simulink library "roller485lib"  (R2023a)
settings: Solver=VariableStepAuto  StartTime=0.0  StopTime=10.0  RelTol=1e-3
libraries: arduinolib x172, simulink x66, $bdroot x1
(part 1 of 5)
settings Model: Creator=kawata  LastModifiedBy=kawata
settings RTWCC: GPUComputeCapability=5.0

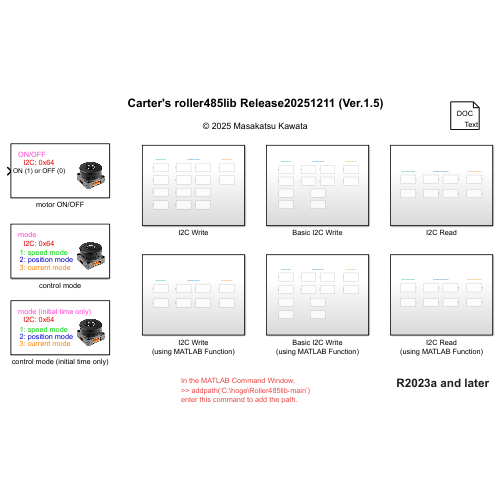
[thumbnail: Simulink's stored preview of the top-level diagram]
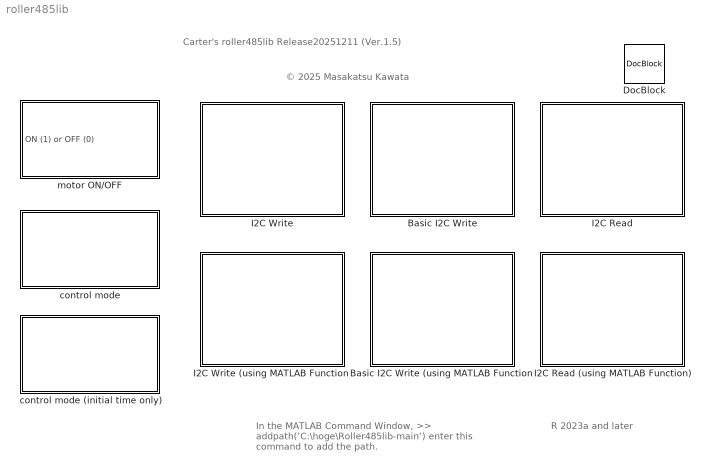
== system roller485lib ==
  note: © 2025 Masakatsu Kawata
  note: Carter's roller485lib Release20251211 (Ver.1.5)
  note: R 2023a and later
  note: In the MATLAB Command Window,
      | >> addpath(‘C:\hoge\Roller485lib-main’)
      | enter this command to add the path.
  Basic I2C Write : Subsystem
  Basic I2C Write (using MATLAB Function) : Subsystem
  DocBlock : simulink/Model-Wide Utilities/DocBlock  DocumentType=Text
      content=|
      | Carter's Roller485lib Ver.1.0
      | Copyright (c) 2025 Masakatsu Kawata
      | Released under the MIT License.
      | See LICENSE for details.
  I2C Read : Subsystem
  I2C Read (using MATLAB Function) : Subsystem
  I2C Write : Subsystem
  I2C Write (using MATLAB Function) : Subsystem
  control mode : Subsystem  mask{I2CAddress=0x64, control_mode=1}
      mask prompts: I2CAddress "I2C Address"; control_mode "mode"
      mask help:
      | 1: speed mode (default)
      | 2: position mode
      | 3: current mode
      | 4: encoder mode
      mask DialogControl ParameterGroupVar Prompt: パラメーター
      mask Display:
      | image('roller485.png', [55,10,75,56]);
      | color('magenta');
      | text(10, 60, 'mode');
      | color('green');
      | text(12, 35, '1: speed mode');
      | color('blue');
      | text(12, 25, '2: position mode');
      | color('orange');
      | text(12, 15, '3: current mode');
      | 
      | color('red');
      | addr = get_param(gcb, 'I2CAddress');
      | text(17, 48, ['I2C: ' addr]);
  control mode (initial time only) : Subsystem  mask{I2CAddress=0x64, control_mode=1}
      mask prompts: I2CAddress "I2C Address"; control_mode "mode"
      mask help:
      | 1: speed mode (default)
      | 2: position mode
      | 3: current mode
      | 4: encoder mode
      | ---------------------------------
      | valid only at the initial time
      mask DialogControl ParameterGroupVar Prompt: パラメーター
      mask Display:
      | image('roller485.png', [55,10,75,56]);
      | color('magenta');
      | text(10, 60, 'mode (initial time only)');
      | color('green');
      | text(12, 35, '1: speed mode');
      | color('blue');
      | text(12, 25, '2: position mode');
      | color('orange');
      | text(12, 15, '3: current mode');
      | 
      | color('red');
      | addr = get_param(gcb, 'I2CAddress');
      | text(17, 48, ['I2C: ' addr]);
  motor ON/OFF : Subsystem  mask{I2CAddress=0x64}
      mask prompts: I2CAddress "I2C Address"
      mask help:
      | 0: motor off
      | 1: motor on
      mask DialogControl ParameterGroupVar Prompt: パラメーター
      mask Display:
      | image('roller485.png', [55,10,75,56]);
      | color('magenta');
      | text(10, 60, 'ON/OFF');
      | 
      | color('red');
      | addr = get_param(gcb, 'I2CAddress');
      | text(17, 48, ['I2C: ' addr]);

== system roller485lib/Basic I2C Write ==
  note: speed mode
  note: current mode
  note: position mode
  basic absolute angle command [deg] : Subsystem  mask{I2CAddress=0x64}
      mask prompts: I2CAddress "I2C Address"
      mask DialogControl ParameterGroupVar Prompt: パラメーター
      mask Display:
      | image('roller485.png', [55,10,75,56]);
      | color('blue');
      | text(10, 60, 'absolute position control');
      | 
      | color('red');
      | addr = get_param(gcb, 'I2CAddress');
      | text(17, 48, ['I2C: ' addr]);
  basic absolute angle command [rad] : Subsystem  mask{I2CAddress=0x64}
      mask prompts: I2CAddress "I2C Address"
      mask DialogControl ParameterGroupVar Prompt: パラメーター
      mask Display:
      | image('roller485.png', [55,10,75,56]);
      | color('blue');
      | text(10, 60, 'absolute position control');
      | 
      | color('red');
      | addr = get_param(gcb, 'I2CAddress');
      | text(17, 48, ['I2C: ' addr]);
  basic angular velocity command [rad/s] : Subsystem  mask{I2CAddress=0x64}
      mask prompts: I2CAddress "I2C Address"
      mask DialogControl ParameterGroupVar Prompt: パラメーター
      mask Display:
      | image('roller485.png', [55,10,75,56]);
      | color('green');
      | text(10, 60, 'speed control');
      | 
      | color('red');
      | addr = get_param(gcb, 'I2CAddress');
      | text(17, 48, ['I2C: ' addr]);
  basic angular velocity command [rpm] : Subsystem  mask{I2CAddress=0x64}
      mask prompts: I2CAddress "I2C Address"
      mask DialogControl ParameterGroupVar Prompt: パラメーター
      mask Display:
      | image('roller485.png', [55,10,75,56]);
      | color('green');
      | text(10, 60, 'speed control');
      | 
      | color('red');
      | addr = get_param(gcb, 'I2CAddress');
      | text(17, 48, ['I2C: ' addr]);
  basic current command [A] : Subsystem  mask{I2CAddress=0x64}
      mask prompts: I2CAddress "I2C Address"
      mask DialogControl ParameterGroupVar Prompt: パラメーター
      mask Display:
      | image('roller485.png', [55,10,75,56]);
      | color('orange');
      | text(10, 60, 'current control');
      | 
      | color('red');
      | addr = get_param(gcb, 'I2CAddress');
      | text(17, 48, ['I2C: ' addr]);
  basic current command [mA] : Subsystem  mask{I2CAddress=0x64}
      mask prompts: I2CAddress "I2C Address"
      mask DialogControl ParameterGroupVar Prompt: パラメーター
      mask Display:
      | image('roller485.png', [55,10,75,56]);
      | color('orange');
      | text(10, 60, 'current control');
      | 
      | color('red');
      | addr = get_param(gcb, 'I2CAddress');
      | text(17, 48, ['I2C: ' addr]);
  basic relative angle command [deg] : Subsystem  mask{I2CAddress=0x64, sample_time=0.005}
      mask prompts: I2CAddress "I2C Address"; sample_time "Sample Time"
      mask DialogControl ParameterGroupVar Prompt: パラメーター
      mask Display:
      | image('roller485.png', [55,10,75,56]);
      | color('blue');
      | text(10, 60, 'relative position control');
      | 
      | color('red');
      | addr = get_param(gcb, 'I2CAddress');
      | text(17, 48, ['I2C: ' addr]);
  basic relative angle command [rad] : Subsystem  mask{I2CAddress=0x64, sample_time=0.005}
      mask prompts: I2CAddress "I2C Address"; sample_time "Sample Time"
      mask DialogControl ParameterGroupVar Prompt: パラメーター
      mask Display:
      | image('roller485.png', [55,10,75,56]);
      | color('blue');
      | text(10, 60, 'relative position control');
      | 
      | color('red');
      | addr = get_param(gcb, 'I2CAddress');
      | text(17, 48, ['I2C: ' addr]);
  position PID : Subsystem  mask{I2CAddress=0x64, position_P=15, position_I=0.000003, position_D=400}
      mask prompts: I2CAddress "I2C Address"; position_P "P"; position_I "I"; position_D "D"
      mask help:
      | position mode
      | ---------------------------------
      | default value
      |  P: 15
      |  I: 0.000003
      |  D: 400
      mask DialogControl ParameterGroupVar Prompt: パラメーター
      mask Display:
      | image('roller485.png', [55,10,75,56]);
      | color('blue');
      | text(10, 60, 'position PID');
      | 
      | color('red');
      | addr = get_param(gcb, 'I2CAddress');
      | text(17, 48, ['I2C: ' addr]);
  position PID (within set time) : Subsystem  mask{I2CAddress=0x64, set_time=0, position_P=15, position_I=0.000003, position_D=400}
      mask prompts: I2CAddress "I2C Address"; set_time "Set Time"; position_P "P"; position_I "I"; position_D "D"
      mask help:
      | position mode
      | ---------------------------------
      | default value
      |  P: 15
      |  I: 0.000003
      |  D: 400
      | ---------------------------------
      | If t ≤ set_time, then PID gain can be set.
      mask DialogControl ParameterGroupVar Prompt: パラメーター
      mask Display:
      | image('roller485.png', [55,10,75,56]);
      | color('blue');
      | text(10, 60, 'position PID');
      | text(10, 47, '(within set time)');
      | 
      | color('red');
      | addr = get_param(gcb, 'I2CAddress');
      | text(17, 34, ['I2C: ' addr]);
  speed PID : Subsystem  mask{I2CAddress=0x64, speed_P=15, speed_I=0.0001, speed_D=400}
      mask prompts: I2CAddress "I2C Address"; speed_P "P"; speed_I "I"; speed_D "D"
      mask help:
      | speed mode
      | ---------------------------------
      | default value
      |  P: 15
      |  I: 0.0001
      |  D: 400
      mask DialogControl ParameterGroupVar Prompt: パラメーター
      mask Display:
      | image('roller485.png', [55,10,75,56]);
      | color('green');
      | text(10, 60, 'speed PID');
      | 
      | color('red');
      | addr = get_param(gcb, 'I2CAddress');
      | text(17, 48, ['I2C: ' addr]);
  speed PID (within set time) : Subsystem  mask{I2CAddress=0x64, set_time=0, speed_P=15, speed_I=0.0001, speed_D=400}
      mask prompts: I2CAddress "I2C Address"; set_time "Set Time"; speed_P "P"; speed_I "I"; speed_D "D"
      mask help:
      | speed mode
      | ---------------------------------
      | default value
      |  P: 15
      |  I: 0.0001
      |  D: 400
      | ---------------------------------
      | valid only at the initial time
      | ---------------------------------
      | If t ≤ set_time, then PID gain can be set.
      mask DialogControl ParameterGroupVar Prompt: パラメーター
      mask Display:
      | image('roller485.png', [55,10,75,56]);
      | color('green');
      | text(10, 60, 'speed PID');
      | text(10, 47, '(within set time)');
      | 
      | color('red');
      | addr = get_param(gcb, 'I2CAddress');
      | text(17, 34, ['I2C: ' addr]);

== system roller485lib/Basic I2C Write (using MATLAB Function) ==
  note: position mode
  note: current mode
  note: speed mode
  basic absolute angle command [deg] (using MATLAB Function) : Subsystem  mask{I2CAddress=0x64}
      mask prompts: I2CAddress "I2C Address"
      mask DialogControl ParameterGroupVar Prompt: パラメーター
      mask Display:
      | image('roller485_matlab_fcn.png', [55,10,75,56]);
      | color('blue');
      | text(10, 60, 'absolute position control');
      | 
      | color('red');
      | addr = get_param(gcb, 'I2CAddress');
      | text(17, 48, ['I2C: ' addr]);
  basic absolute angle command [rad] (using MATLAB Function) : Subsystem  mask{I2CAddress=0x64}
      mask prompts: I2CAddress "I2C Address"
      mask DialogControl ParameterGroupVar Prompt: パラメーター
      mask Display:
      | image('roller485_matlab_fcn.png', [55,10,75,56]);
      | color('blue');
      | text(10, 60, 'absolute position control');
      | 
      | color('red');
      | addr = get_param(gcb, 'I2CAddress');
      | text(17, 48, ['I2C: ' addr]);
  basic angular velocity command [rad/s] (using MATLAB Function) : Subsystem  mask{I2CAddress=0x64}
      mask prompts: I2CAddress "I2C Address"
      mask DialogControl ParameterGroupVar Prompt: パラメーター
      mask Display:
      | image('roller485_matlab_fcn.png', [55,10,75,56]);
      | color('green');
      | text(10, 60, 'speed control');
      | 
      | color('red');
      | addr = get_param(gcb, 'I2CAddress');
      | text(17, 48, ['I2C: ' addr]);
  basic angular velocity command [rpm] (using MATLAB Function) : Subsystem  mask{I2CAddress=0x64}
      mask prompts: I2CAddress "I2C Address"
      mask DialogControl ParameterGroupVar Prompt: パラメーター
      mask Display:
      | image('roller485_matlab_fcn.png', [55,10,75,56]);
      | color('green');
      | text(10, 60, 'speed control');
      | 
      | color('red');
      | addr = get_param(gcb, 'I2CAddress');
      | text(17, 48, ['I2C: ' addr]);
  basic current command [A] (using MATLAB Function) : Subsystem  mask{I2CAddress=0x64}
      mask prompts: I2CAddress "I2C Address"
      mask DialogControl ParameterGroupVar Prompt: パラメーター
      mask Display:
      | image('roller485_matlab_fcn.png', [55,10,75,56]);
      | color('orange');
      | text(10, 60, 'current control');
      | 
      | color('red');
      | addr = get_param(gcb, 'I2CAddress');
      | text(17, 48, ['I2C: ' addr]);
  basic current command [mA] (using MATLAB Function) : Subsystem  mask{I2CAddress=0x64}
      mask prompts: I2CAddress "I2C Address"
      mask DialogControl ParameterGroupVar Prompt: パラメーター
      mask Display:
      | image('roller485_matlab_fcn.png', [55,10,75,56]);
      | color('orange');
      | text(10, 60, 'current control');
      | 
      | color('red');
      | addr = get_param(gcb, 'I2CAddress');
      | text(17, 48, ['I2C: ' addr]);
  basic relative angle command [deg] (using MATLAB Function) : Subsystem  mask{I2CAddress=0x64, sample_time=0.005}
      mask prompts: I2CAddress "I2C Address"; sample_time "Sample Time"
      mask DialogControl ParameterGroupVar Prompt: パラメーター
      mask Display:
      | image('roller485_matlab_fcn.png', [55,10,75,56]);
      | color('blue');
      | text(10, 60, 'relative position control');
      | 
      | color('red');
      | addr = get_param(gcb, 'I2CAddress');
      | text(17, 48, ['I2C: ' addr]);
  basic relative angle command [rad] (using MATLAB Function) : Subsystem  mask{I2CAddress=0x64, sample_time=0.005}
      mask prompts: I2CAddress "I2C Address"; sample_time "Sample Time"
      mask DialogControl ParameterGroupVar Prompt: パラメーター
      mask Display:
      | image('roller485_matlab_fcn.png', [55,10,75,56]);
      | color('blue');
      | text(10, 60, 'relative position control');
      | 
      | color('red');
      | addr = get_param(gcb, 'I2CAddress');
      | text(17, 48, ['I2C: ' addr]);
  position PID (using MATLAB Function) : Subsystem  mask{I2CAddress=0x64, position_P=15, position_I=0.000003, position_D=400}
      mask prompts: I2CAddress "I2C Address"; position_P "P"; position_I "I"; position_D "D"
      mask help:
      | position mode
      | ---------------------------------
      | default value
      |  P: 15
      |  I: 0.000003
      |  D: 400
      mask DialogControl ParameterGroupVar Prompt: パラメーター
      mask Display:
      | image('roller485_matlab_fcn.png', [55,10,75,56]);
      | color('blue');
      | text(10, 60, 'position PID');
      | 
      | color('red');
      | addr = get_param(gcb, 'I2CAddress');
      | text(17, 48, ['I2C: ' addr]);
  position PID (within set time) (using MATLAB Function) : Subsystem  mask{I2CAddress=0x64, set_time=0, position_P=15, position_I=0.000003, position_D=400}
      mask prompts: I2CAddress "I2C Address"; set_time "Set Time"; position_P "P"; position_I "I"; position_D "D"
      mask help:
      | position mode
      | ---------------------------------
      | default value
      |  P: 15
      |  I: 0.000003
      |  D: 400
      | ---------------------------------
      | If t ≤ set_time, then PID gain can be set.
      mask DialogControl ParameterGroupVar Prompt: パラメーター
      mask Display:
      | image('roller485_matlab_fcn.png', [55,10,75,56]);
      | color('blue');
      | text(10, 60, 'position PID');
      | text(10, 47, '(within set time)');
      | 
      | color('red');
      | addr = get_param(gcb, 'I2CAddress');
      | text(17, 34, ['I2C: ' addr]);
  speed PID (using MATLAB Function) : Subsystem  mask{I2CAddress=0x64, speed_P=15, speed_I=0.0001, speed_D=400}
      mask prompts: I2CAddress "I2C Address"; speed_P "P"; speed_I "I"; speed_D "D"
      mask help:
      | speed mode
      | ---------------------------------
      | default value
      |  P: 15
      |  I: 0.0001
      |  D: 400
      mask DialogControl ParameterGroupVar Prompt: パラメーター
      mask Display:
      | image('roller485_matlab_fcn.png', [55,10,75,56]);
      | color('green');
      | text(10, 60, 'speed PID');
      | 
      | color('red');
      | addr = get_param(gcb, 'I2CAddress');
      | text(17, 48, ['I2C: ' addr]);
  speed PID (within set time) (using MATLAB Function) : Subsystem  mask{I2CAddress=0x64, set_time=0, speed_P=15, speed_I=0.0001, speed_D=400}
      mask prompts: I2CAddress "I2C Address"; set_time "Set Time"; speed_P "P"; speed_I "I"; speed_D "D"
      mask help:
      | speed mode
      | ---------------------------------
      | default value
      |  P: 15
      |  I: 0.0001
      |  D: 400
      | ---------------------------------
      | If t ≤ set_time, then PID gain can be set.
      mask DialogControl ParameterGroupVar Prompt: パラメーター
      mask Display:
      | image('roller485_matlab_fcn.png', [55,10,75,56]);
      | color('green');
      | text(10, 60, 'speed PID');
      | text(10, 47, '(within set time)');
      | 
      | color('red');
      | addr = get_param(gcb, 'I2CAddress');
      | text(17, 34, ['I2C: ' addr]);

== system roller485lib/I2C Read ==
  note: speed detection
  note: current detection
  note: position detection
  absolute angle detection [deg] : Subsystem  mask{I2CAddress=0x64, sample_time=0.005}
      mask prompts: I2CAddress "I2C Address"; sample_time "Sample Time"
      mask DialogControl ParameterGroupVar Prompt: パラメーター
      mask Display:
      | image('roller485.png', [30,10,75,56]);
      | color('blue');
      | text(10, 60, 'absolute angle detection');
      | 
      | color('red');
      | addr = get_param(gcb, 'I2CAddress');
      | text(17, 48, ['I2C: ' addr]);
  absolute angle detection [rad] : Subsystem  mask{I2CAddress=0x64, sample_time=0.005}
      mask prompts: I2CAddress "I2C Address"; sample_time "Sample Time"
      mask DialogControl ParameterGroupVar Prompt: パラメーター
      mask Display:
      | image('roller485.png', [30,10,75,56]);
      | color('blue');
      | text(10, 60, 'absolute angle detection');
      | 
      | color('red');
      | addr = get_param(gcb, 'I2CAddress');
      | text(17, 48, ['I2C: ' addr]);
  angular velocity detection using LPF [rad/s] : Subsystem  mask{I2CAddress=0x64, sample_time=0.005}
      mask prompts: I2CAddress "I2C Address"; sample_time "Sample Time"
      mask DialogControl ParameterGroupVar Prompt: パラメーター
      mask Display:
      | image('roller485.png', [30,10,75,56]);
      | color('green');
      | text(10, 60, 'speed detection');
      | 
      | color('red');
      | addr = get_param(gcb, 'I2CAddress');
      | text(17, 48, ['I2C: ' addr]);
  angular velocity detection using LPF [rpm] : Subsystem  mask{I2CAddress=0x64, sample_time=0.005}
      mask prompts: I2CAddress "I2C Address"; sample_time "Sample Time"
      mask DialogControl ParameterGroupVar Prompt: パラメーター
      mask Display:
      | image('roller485.png', [30,10,75,56]);
      | color('green');
      | text(10, 60, 'speed detection');
      | 
      | color('red');
      | addr = get_param(gcb, 'I2CAddress');
      | text(17, 48, ['I2C: ' addr]);
  current detection [A] : Subsystem  mask{I2CAddress=0x64, sample_time=0.005}
      mask prompts: I2CAddress "I2C Address"; sample_time "Sample Time"
      mask DialogControl ParameterGroupVar Prompt: パラメーター
      mask Display:
      | image('roller485.png', [30,10,75,56]);
      | color('orange');
      | text(10, 60, 'current detection');
      | 
      | color('red');
      | addr = get_param(gcb, 'I2CAddress');
      | text(17, 48, ['I2C: ' addr]);
  current detection [mA] : Subsystem  mask{I2CAddress=0x64, sample_time=0.005}
      mask prompts: I2CAddress "I2C Address"; sample_time "Sample Time"
      mask DialogControl ParameterGroupVar Prompt: パラメーター
      mask Display:
      | image('roller485.png', [30,10,75,56]);
      | color('orange');
      | text(10, 60, 'current detection');
      | 
      | color('red');
      | addr = get_param(gcb, 'I2CAddress');
      | text(17, 48, ['I2C: ' addr]);
  relative angle detection [deg] : Subsystem  mask{I2CAddress=0x64, sample_time=0.005, set_time=0}
      mask prompts: I2CAddress "I2C Address"; sample_time "Sample Time"; set_time "Set Time"
      mask help: If t ≤ set_time, then initial angle is set.
      mask DialogControl ParameterGroupVar Prompt: パラメーター
      mask Display:
      | image('roller485.png', [30,10,75,56]);
      | color('blue');
      | text(10, 60, 'relative angle detection');
      | 
      | color('red');
      | addr = get_param(gcb, 'I2CAddress');
      | text(17, 48, ['I2C: ' addr]);
  relative angle detection [rad] : Subsystem  mask{I2CAddress=0x64, sample_time=0.005, set_time=0}
      mask prompts: I2CAddress "I2C Address"; sample_time "Sample Time"; set_time "Set Time"
      mask help: If t ≤ set_time, then initial angle is set.
      mask DialogControl ParameterGroupVar Prompt: パラメーター
      mask Display:
      | image('roller485.png', [30,10,75,56]);
      | color('blue');
      | text(10, 60, 'relative angle detection');
      | 
      | color('red');
      | addr = get_param(gcb, 'I2CAddress');
      | text(17, 48, ['I2C: ' addr]);

== system roller485lib/I2C Read (using MATLAB Function) ==
  note: position detection
  note: current detection
  note: speed detection
  absolute angle detection [deg] (using MATLAB Function) : Subsystem  mask{I2CAddress=0x64, sample_time=0.005}
      mask prompts: I2CAddress "I2C Address"; sample_time "Sample Time"
      mask DialogControl ParameterGroupVar Prompt: パラメーター
      mask Display:
      | image('roller485_matlab_fcn.png', [38,10,75,56]);
      | color('blue');
      | text(10, 60, 'absolute angle detection');
      | 
      | color('red');
      | addr = get_param(gcb, 'I2CAddress');
      | text(17, 48, ['I2C: ' addr]);
  absolute angle detection [rad] (using MATLAB Function) : Subsystem  mask{I2CAddress=0x64, sample_time=0.005}
      mask prompts: I2CAddress "I2C Address"; sample_time "Sample Time"
      mask DialogControl ParameterGroupVar Prompt: パラメーター
      mask Display:
      | image('roller485_matlab_fcn.png', [38,10,75,56]);
      | color('blue');
      | text(10, 60, 'absolute angle detection');
      | 
      | color('red');
      | addr = get_param(gcb, 'I2CAddress');
      | text(17, 48, ['I2C: ' addr]);
  angular velocity detection using LPF [rad/s] (using MATLAB Function) : Subsystem  mask{I2CAddress=0x64, sample_time=0.005}
      mask prompts: I2CAddress "I2C Address"; sample_time "Sample Time"
      mask DialogControl ParameterGroupVar Prompt: パラメーター
      mask Display:
      | image('roller485_matlab_fcn.png', [38,10,75,56]);
      | color('green');
      | text(10, 60, 'speed detection');
      | 
      | color('red');
      | addr = get_param(gcb, 'I2CAddress');
      | text(17, 48, ['I2C: ' addr]);
  angular velocity detection using LPF [rpm] (using MATLAB Function) : Subsystem  mask{I2CAddress=0x64, sample_time=0.005}
      mask prompts: I2CAddress "I2C Address"; sample_time "Sample Time"
      mask DialogControl ParameterGroupVar Prompt: パラメーター
      mask Display:
      | image('roller485_matlab_fcn.png', [38,10,75,56]);
      | color('green');
      | text(10, 60, 'speed detection');
      | 
      | color('red');
      | addr = get_param(gcb, 'I2CAddress');
      | text(17, 48, ['I2C: ' addr]);
  current detection [A] (using MATLAB Function) : Subsystem  mask{I2CAddress=0x64, sample_time=0.005}
      mask prompts: I2CAddress "I2C Address"; sample_time "Sample Time"
      mask DialogControl ParameterGroupVar Prompt: パラメーター
      mask Display:
      | image('roller485_matlab_fcn.png', [38,10,75,56]);
      | color('orange');
      | text(10, 60, 'current detection');
      | 
      | color('red');
      | addr = get_param(gcb, 'I2CAddress');
      | text(17, 48, ['I2C: ' addr]);
  current detection [mA] (using MATLAB Function) : Subsystem  mask{I2CAddress=0x64, sample_time=0.005}
      mask prompts: I2CAddress "I2C Address"; sample_time "Sample Time"
      mask DialogControl ParameterGroupVar Prompt: パラメーター
      mask Display:
      | image('roller485_matlab_fcn.png', [38,10,75,56]);
      | color('orange');
      | text(10, 60, 'current detection');
      | 
      | color('red');
      | addr = get_param(gcb, 'I2CAddress');
      | text(17, 48, ['I2C: ' addr]);
  relative angle detection [deg] (using MATLAB Function) : Subsystem  mask{I2CAddress=0x64, sample_time=0.005, set_time=0}
      mask prompts: I2CAddress "I2C Address"; sample_time "Sample Time"; set_time "Set Time"
      mask help: If t ≤ set_time, then initial angle is set.
      mask DialogControl ParameterGroupVar Prompt: パラメーター
      mask Display:
      | image('roller485_matlab_fcn.png', [38,10,75,56]);
      | color('blue');
      | text(10, 60, 'relative angle detection');
      | 
      | color('red');
      | addr = get_param(gcb, 'I2CAddress');
      | text(17, 48, ['I2C: ' addr]);
  relative angle detection [rad] (using MATLAB Function) : Subsystem  mask{I2CAddress=0x64, sample_time=0.005, set_time=0}
      mask prompts: I2CAddress "I2C Address"; sample_time "Sample Time"; set_time "Set Time"
      mask help: If t ≤ set_time, then initial angle is set.
      mask DialogControl ParameterGroupVar Prompt: パラメーター
      mask Display:
      | image('roller485_matlab_fcn.png', [38,10,75,56]);
      | color('blue');
      | text(10, 60, 'relative angle detection');
      | 
      | color('red');
      | addr = get_param(gcb, 'I2CAddress');
      | text(17, 48, ['I2C: ' addr]);

== system roller485lib/I2C Write ==
  note: position mode
  note: current mode
  note: speed mode
  absolute angle command [deg] : Subsystem  mask(absolute angle command [deg]){I2CAddress=0x64, position_P=15, position_I=0.000003, position_D=400, set_time1=0, set_time2=0}
      mask prompts: I2CAddress "I2C Address"; position_P "P"; position_I "I"; position_D "D"; set_time1 "Set Time1"; set_time2 "Set Time2"
      mask help:
      | position mode
      | If t ≤ set_time1, then position mode is set.
      | ---------------------------------
      | default value (PID gain of position controller)
      |  P: 15
      |  I: 0.000003
      |  D: 400
      | If t ≤ set_time2, then PID gain can be set.
      mask DialogControl ParameterGroupVar Prompt: パラメーター
      mask Display:
      | image('roller485.png', [55,10,75,56]);
      | color('blue');
      | text(10, 60, 'absolute position control');
      | text(17, 22, '# mode setting');
      | text(17, 10, '# PID gain setting');
      | color('black');
      | 
      | color('red');
      | addr = get_param(gcb, 'I2CAddress');
      | text(17, 48, ['I2C: ' addr]);
  absolute angle command [deg] and max current [mA] : Subsystem  mask(absolute angle command [deg]){I2CAddress=0x64, position_P=15, position_I=0.000003, position_D=400, max_current=1000, set_time1=0, set_time2=0, set_time3=0}
      mask prompts: I2CAddress "I2C Address"; position_P "P"; position_I "I"; position_D "D"; max_current "Imax [mA]"; set_time1 "Set Time1"; set_time2 "Set Time2"; set_time3 "Set Time3"
      mask help:
      | position mode
      | If t ≤ set_time1, then position mode is set.
      | ---------------------------------
      | default value (PID gain of position controller)
      |  P: 15
      |  I: 0.000003
      |  D: 400
      | If t ≤ set_time2, then PID gain can be set.
      | ---------------------------------
      | default value (Imax: max current)
      |  Imax: 1000 mA
      |   ---> Imax can be set up to a maximum of 1200mA.
      | If t ≤ set_time3, then Imax can be set.
      mask DialogControl ParameterGroupVar Prompt: パラメーター
      mask Display:
      | image('roller485.png', [55,10,75,56]);
      | color('blue');
      | text(10, 60, 'absolute position control');
      | text(17, 22, '# mode setting');
      | text(17, 10, '# PID gain & Imax setting');
      | 
      | color('red');
      | addr = get_param(gcb, 'I2CAddress');
      | text(17, 48, ['I2C: ' addr]);
  absolute angle command [rad] : Subsystem  mask(absolute angle command [rad]){I2CAddress=0x64, position_P=15, position_I=0.000003, position_D=400, set_time1=0, set_time2=0}
      mask prompts: I2CAddress "I2C Address"; position_P "P"; position_I "I"; position_D "D"; set_time1 "Set Time1"; set_time2 "Set Time2"
      mask help:
      | position mode
      | If t ≤ set_time1, then position mode is set.
      | ---------------------------------
      | default value (PID gain of position controller)
      |  P: 15
      |  I: 0.000003
      |  D: 400
      | If t ≤ set_time2, then PID gain can be set.
      mask DialogControl ParameterGroupVar Prompt: パラメーター
      mask Display:
      | image('roller485.png', [55,10,75,56]);
      | color('blue');
      | text(10, 60, 'absolute position control');
      | text(17, 22, '# mode setting');
      | text(17, 10, '# PID gain setting');
      | 
      | color('red');
      | addr = get_param(gcb, 'I2CAddress');
      | text(17, 48, ['I2C: ' addr]);
  absolute angle command [rad] and max current [mA] : Subsystem  mask(absolute angle command [rad]){I2CAddress=0x64, position_P=15, position_I=0.000003, position_D=400, max_current=1000, set_time1=0, set_time2=0, set_time3=0}
      mask prompts: I2CAddress "I2C Address"; position_P "P"; position_I "I"; position_D "D"; max_current "Imax [mA]"; set_time1 "Set Time1"; set_time2 "Set Time2"; set_time3 "Set Time3"
      mask help:
      | position mode
      | If t ≤ set_time1, then position mode is set.
      | ---------------------------------
      | default value (PID gain of position controller)
      |  P: 15
      |  I: 0.000003
      |  D: 400
      | If t ≤ set_time2, then PID gain can be set.
      | ---------------------------------
      | default value (Imax: max current)
      |  Imax: 1000 mA
      |   ---> Imax can be set up to a maximum of 1200mA.
      | If t ≤ set_time3, then Imax can be set.
      mask DialogControl ParameterGroupVar Prompt: パラメーター
      mask Display:
      | image('roller485.png', [55,10,75,56]);
      | color('blue');
      | text(10, 60, 'absolute position control');
      | text(17, 22, '# mode setting');
      | text(17, 10, '# PID gain & Imax setting');
      | 
      | color('red');
      | addr = get_param(gcb, 'I2CAddress');
      | text(17, 48, ['I2C: ' addr]);
  angular velocity command [rad/s] : Subsystem  mask(angular velocity command [rad/s]){I2CAddress=0x64, speed_P=15, speed_I=0.0001, speed_D=400, set_time1=0, set_time2=0}
      mask prompts: I2CAddress "I2C Address"; speed_P "P"; speed_I "I"; speed_D "D"; set_time1 "Set Time1"; set_time2 "Set Time2"
      mask help:
      | speed mode
      | If t ≤ set_time1, then speed mode is set.
      | ---------------------------------
      | default value (PID gain of speed controller)
      |  P: 15
      |  I: 0.0001
      |  D: 400
      | If t ≤ set_time2, then PID gain can be set.
      mask DialogControl ParameterGroupVar Prompt: パラメーター
      mask Display:
      | image('roller485.png', [55,10,75,56]);
      | color('green');
      | text(10, 60, 'speed control');
      | text(17, 22, '# mode setting');
      | text(17, 10, '# PID gain setting');
      | 
      | color('red');
      | addr = get_param(gcb, 'I2CAddress');
      | text(17, 48, ['I2C: ' addr]);
  angular velocity command [rad/s] and max current [mA] : Subsystem  mask(angular velocity command [rad/s]){I2CAddress=0x64, speed_P=15, speed_I=0.0001, speed_D=400, max_current=1000, set_time1=0, set_time2=0, set_time3=0}
      mask prompts: I2CAddress "I2C Address"; speed_P "P"; speed_I "I"; speed_D "D"; max_current "Imax [mA]"; set_time1 "Set Time1"; set_time2 "Set Time2"; set_time3 "Set Time3"
      mask help:
      | speed mode
      | If t ≤ set_time1, then speed mode is set.
      | ---------------------------------
      | default value (PID gain of speed controller)
      |  P: 15
      |  I: 0.0001
      |  D: 400
      | If t ≤ set_time2, then PID gain and Imax can be set.
      | ---------------------------------
      | default value (Imax: max current)
      |  Imax: 1000 mA
      |  ---> Imax can be set up to a maximum of 1200mA.
      | If t ≤ set_time3, then Imax is set.
      mask DialogControl ParameterGroupVar Prompt: パラメーター
      mask Display:
      | image('roller485.png', [55,10,75,56]);
      | color('green');
      | text(10, 60, 'speed control');
      | text(17, 22, '# mode setting');
      | text(17, 10, '# PID gain & Imax setting');
      | 
      | color('red');
      | addr = get_param(gcb, 'I2CAddress');
      | text(17, 48, ['I2C: ' addr]);
  angular velocity command [rpm] : Subsystem  mask(angular velocity command [rpm]){I2CAddress=0x64, speed_P=15, speed_I=0.0001, speed_D=400, set_time1=0, set_time2=0}
      mask prompts: I2CAddress "I2C Address"; speed_P "P"; speed_I "I"; speed_D "D"; set_time1 "Set Time1"; set_time2 "Set Time2"
      mask help:
      | speed mode
      | If t ≤ set_time1, then speed mode is set.
      | ---------------------------------
      | default value (PID gain of speed controller)
      |  P: 15
      |  I: 0.0001
      |  D: 400
      | If t ≤ set_time2, then PID gain can be set.
      mask DialogControl ParameterGroupVar Prompt: パラメーター
      mask Display:
      | image('roller485.png', [55,10,75,56]);
      | color('green');
      | text(10, 60, 'speed control');
      | color('green');
      | text(17, 22, '# mode setting');
      | text(17, 10, '# PID gain setting');
      | 
      | color('red');
      | addr = get_param(gcb, 'I2CAddress');
      | text(17, 48, ['I2C: ' addr]);
  angular velocity command [rpm] and max current [mA] : Subsystem  mask(angular velocity command [rpm]){I2CAddress=0x64, speed_P=15, speed_I=0.0001, speed_D=400, max_current=1000, set_time1=0, set_time2=0, set_time3=0}
      mask prompts: I2CAddress "I2C Address"; speed_P "P"; speed_I "I"; speed_D "D"; max_current "Imax [mA]"; set_time1 "Set Time1"; set_time2 "Set Time2"; set_time3 "Set Time3"
      mask help:
      | speed mode
      | If t ≤ set_time1, then speed mode is set.
      | ---------------------------------
      | default value (PID gain of speed controller)
      |  P: 15
      |  I: 0.0001
      |  D: 400
      | If t ≤ set_time2, then PID gain and Imax can be set.
      | ---------------------------------
      | default value (Imax: max current)
      |  Imax: 1000 mA
      |  ---> Imax can be set up to a maximum of 1200mA.
      | If t ≤ set_time3, then Imax is set.
      mask DialogControl ParameterGroupVar Prompt: パラメーター
      mask Display:
      | image('roller485.png', [55,10,75,56]);
      | color('green');
      | text(10, 60, 'speed control');
      | text(17, 22, '# mode setting');
      | text(17, 10, '# PID gain & Imax setting');
      | 
      | color('red');
      | addr = get_param(gcb, 'I2CAddress');
      | text(17, 48, ['I2C: ' addr]);
  current command [A] : Subsystem  mask(current command [A]){I2CAddress=0x64, set_time=0}
      mask prompts: I2CAddress "I2C Address"; set_time "Set Time"
      mask help:
      | current mode
      | If t ≤ set_time, then current mode is set.
      | ---------------------------------
      | PID gain of current controller
      |  P: 0.002
      |  I: 0.00005
      |  D: 0
      | Changing the PID gains is not permitted.
      mask DialogControl ParameterGroupVar Prompt: パラメーター
      mask Display:
      | image('roller485.png', [55,10,75,56]);
      | color('orange');
      | text(10, 60, 'current control');
      | text(17, 22, '# mode setting');
      | 
      | color('red');
      | addr = get_param(gcb, 'I2CAddress');
      | text(17, 48, ['I2C: ' addr]);
  current command [mA] : Subsystem  mask(current command [A]){I2CAddress=0x64, set_time=0}
      mask prompts: I2CAddress "I2C Address"; set_time "Set Time"
      mask help:
      | current mode
      | If t ≤ set_time, then current mode is set.
      | ---------------------------------
      | PID gain of current controller
      |  P: 0.002
      |  I: 0.00005
      |  D: 0
      | Changing the PID gains is not permitted.
      mask DialogControl ParameterGroupVar Prompt: パラメーター
      mask Display:
      | image('roller485.png', [55,10,75,56]);
      | color('orange');
      | text(10, 60, 'current control');
      | text(17, 22, '# mode setting');
      | 
      | color('red');
      | addr = get_param(gcb, 'I2CAddress');
      | text(17, 48, ['I2C: ' addr]);
  relative angle command [deg] : Subsystem  mask(relative angle command [deg]){I2CAddress=0x64, sample_time=0.005, position_P=15, position_I=0.000003, position_D=400, set_time1=0, set_time2=0}
      mask prompts: I2CAddress "I2C Address"; sample_time "Sample Time"; position_P "P"; position_I "I"; position_D "D"; set_time1 "Set Time1"; set_time2 "Set Time2"
      mask help:
      | position mode
      | If t ≤ set_time1, then position mode and initial angle are set.
      | ---------------------------------
      | default value (PID gain of position controller)
      |  P: 15
      |  I: 0.000003
      |  D: 400
      | If t ≤ set_time2, then PID gain can be set.
      mask DialogControl ParameterGroupVar Prompt: パラメーター
      mask Display:
      | image('roller485.png', [55,10,75,56]);
      | color('blue');
      | text(10, 60, 'relative position control');
      | text(17, 22, '# mode setting');
      | text(17, 10, '# PID gain setting');
      | 
      | color('red');
      | addr = get_param(gcb, 'I2CAddress');
      | text(17, 48, ['I2C: ' addr]);
  relative angle command [deg] and max current [mA] : Subsystem  mask(relative angle command [rad]){I2CAddress=0x64, sample_time=0.005, position_P=15, position_I=0.000003, position_D=400, max_current=1000, set_time1=0, set_time2=0, set_time3=0}
      mask prompts: I2CAddress "I2C Address"; sample_time "Sample Time"; position_P "P"; position_I "I"; position_D "D"; max_current "Imax [mA]"; set_time1 "Set Time1"; set_time2 "Set Time2"; set_time3 "Set Time3"
      mask help:
      | position mode
      | If t ≤ set_time1, then position mode and initial angle are set.
      | ---------------------------------
      | default value (PID gain of position controller)
      |  P: 15
      |  I: 0.000003
      |  D: 400
      | If t ≤ set_time2, then PID gain can be set.
      | ---------------------------------
      | default value (Imax: max current)
      |  Imax: 1000 mA
      |   ---> Imax can be set up to a maximum of 1200mA.
      | If t ≤ set_time3, then Imax can be set.
      mask DialogControl ParameterGroupVar Prompt: パラメーター
      mask Display:
      | image('roller485.png', [55,10,75,56]);
      | color('blue');
      | text(10, 60, 'relative position control');
      | text(17, 22, '# mode setting');
      | text(17, 10, '# PID gain & Imax setting');
      | 
      | color('red');
      | addr = get_param(gcb, 'I2CAddress');
      | text(17, 48, ['I2C: ' addr]);
  relative angle command [rad] : Subsystem  mask(relative angle command [rad]){I2CAddress=0x64, sample_time=0.005, position_P=15, position_I=0.000003, position_D=400, set_time1=0, set_time2=0}
      mask prompts: I2CAddress "I2C Address"; sample_time "Sample Time"; position_P "P"; position_I "I"; position_D "D"; set_time1 "Set Time1"; set_time2 "Set Time2"
      mask help:
      | position mode
      | If t ≤ set_time1, then position mode and initial angle are set.
      | ---------------------------------
      | default value (PID gain of position controller)
      |  P: 15
      |  I: 0.000003
      |  D: 400
      | If t ≤ set_time2, then PID gain can be set.
      mask DialogControl ParameterGroupVar Prompt: パラメーター
      mask Display:
      | image('roller485.png', [55,10,75,56]);
      | color('blue');
      | text(10, 60, 'relative position control');
      | text(17, 22, '# mode setting');
      | text(17, 10, '# PID gain setting');
      | 
      | color('red');
      | addr = get_param(gcb, 'I2CAddress');
      | text(17, 48, ['I2C: ' addr]);
  relative angle command [rad] and max current [mA] : Subsystem  mask(relative angle command [rad]){I2CAddress=0x64, sample_time=0.005, position_P=15, position_I=0.000003, position_D=400, max_current=1000, set_time1=0, set_time2=0, set_time3=0}
      mask prompts: I2CAddress "I2C Address"; sample_time "Sample Time"; position_P "P"; position_I "I"; position_D "D"; max_current "Imax [mA]"; set_time1 "Set Time1"; set_time2 "Set Time2"; set_time3 "Set Time3"
      mask help:
      | position mode
      | If t ≤ set_time1, then position mode and initial angle are set.
      | ---------------------------------
      | default value (PID gain of position controller)
      |  P: 15
      |  I: 0.000003
      |  D: 400
      | If t ≤ set_time2, then PID gain can be set.
      | ---------------------------------
      | default value (Imax: max current)
      |  Imax: 1000 mA
      |   ---> Imax can be set up to a maximum of 1200mA.
      | If t ≤ set_time3, then Imax can be set.
      mask DialogControl ParameterGroupVar Prompt: パラメーター
      mask Display:
      | image('roller485.png', [55,10,75,56]);
      | color('blue');
      | text(10, 60, 'relative position control');
      | text(17, 22, '# mode setting');
      | text(17, 10, '# PID gain & Imax setting');
      | 
      | color('red');
      | addr = get_param(gcb, 'I2CAddress');
      | text(17, 48, ['I2C: ' addr]);

== system roller485lib/I2C Write (using MATLAB Function) ==
  note: speed mode
  note: current mode
  note: position mode
  absolute angle command [deg] (using MATLAB Function) : Subsystem  mask(absolute angle command [deg]){I2CAddress=0x64, position_P=15, position_I=0.000003, position_D=400, set_time1=0, set_time2=0}
      mask prompts: I2CAddress "I2C Address"; position_P "P"; position_I "I"; position_D "D"; set_time1 "Set Time1"; set_time2 "Set Time2"
      mask help:
      | position mode
      | If t ≤ set_time1, then position mode is set.
      | ---------------------------------
      | default value (PID gain of position controller)
      |  P: 15
      |  I: 0.000003
      |  D: 400
      | If t ≤ set_time2, then PID gain can be set.
      mask DialogControl ParameterGroupVar Prompt: パラメーター
      mask Display:
      | image('roller485_matlab_fcn.png', [55,10,75,56]);
      | color('blue');
      | text(10, 60, 'absolute position control');
      | text(17, 22, '# mode setting');
      | text(17, 10, '# PID gain setting');
      | 
      | color('red');
      | addr = get_param(gcb, 'I2CAddress');
      | text(17, 48, ['I2C: ' addr]);
  absolute angle command [rad] (using MATLAB Function) : Subsystem  mask(absolute angle command [rad]){I2CAddress=0x64, position_P=15, position_I=0.000003, position_D=400, set_time1=0, set_time2=0}
      mask prompts: I2CAddress "I2C Address"; position_P "P"; position_I "I"; position_D "D"; set_time1 "Set Time1"; set_time2 "Set Time2"
      mask help:
      | position mode
      | If t ≤ set_time1, then position mode is set.
      | ---------------------------------
      | default value (PID gain of position controller)
      |  P: 15
      |  I: 0.000003
      |  D: 400
      | If t ≤ set_time2, then PID gain can be set.
      mask DialogControl ParameterGroupVar Prompt: パラメーター
      mask Display:
      | image('roller485_matlab_fcn.png', [55,10,75,56]);
      | color('blue');
      | text(10, 60, 'absolute position control');
      | text(17, 22, '# mode setting');
      | text(17, 10, '# PID gain setting');
      | 
      | color('red');
      | addr = get_param(gcb, 'I2CAddress');
      | text(17, 48, ['I2C: ' addr]);
  angular velocity command [rad/s] (using MATLAB Function) : Subsystem  mask(angular velocity command [rad/s]){I2CAddress=0x64, speed_P=15, speed_I=0.0001, speed_D=400, set_time1=0, set_time2=0}
      mask prompts: I2CAddress "I2C Address"; speed_P "P"; speed_I "I"; speed_D "D"; set_time1 "Set Time1"; set_time2 "Set Time2"
      mask help:
      | speed mode
      | If t ≤ set_time1, then speed mode is set.
      | ---------------------------------
      | default value (PID gain of speed controller)
      |  P: 15
      |  I: 0.0001
      |  D: 400
      | If t ≤ set_time2, then PID gain can be set.
      mask DialogControl ParameterGroupVar Prompt: パラメーター
      mask Display:
      | image('roller485_matlab_fcn.png', [55,10,75,56]);
      | color('green');
      | text(10, 60, 'speed control');
      | text(17, 22, '# mode setting');
      | text(17, 10, '# PID gain setting');
      | 
      | color('red');
      | addr = get_param(gcb, 'I2CAddress');
      | text(17, 48, ['I2C: ' addr]);
  angular velocity command [rpm] (using MATLAB Function) : Subsystem  mask(angular velocity command [rpm]){I2CAddress=0x64, speed_P=15, speed_I=0.0001, speed_D=400, set_time1=0, set_time2=0}
      mask prompts: I2CAddress "I2C Address"; speed_P "P"; speed_I "I"; speed_D "D"; set_time1 "Set Time1"; set_time2 "Set Time2"
      mask help:
      | speed mode
      | If t ≤ set_time1, then speed mode is set.
      | ---------------------------------
      | default value (PID gain of speed controller)
      |  P: 15
      |  I: 0.0001
      |  D: 400
      | If t ≤ set_time2, then PID gain can be set.
      mask DialogControl ParameterGroupVar Prompt: パラメーター
      mask Display:
      | image('roller485_matlab_fcn.png', [55,10,75,56]);
      | color('green');
      | text(10, 60, 'speed control');
      | text(17, 22, '# mode setting');
      | text(17, 10, '# PID gain setting');
      | 
      | color('red');
      | addr = get_param(gcb, 'I2CAddress');
      | text(17, 48, ['I2C: ' addr]);
  current command [A] (using MATLAB Function) : Subsystem  mask(current command [A]){I2CAddress=0x64, set_time=0}
      mask prompts: I2CAddress "I2C Address"; set_time "Set Time"
      mask help:
      | current mode
      | If t ≤ set_time, then current mode is set.
      | ---------------------------------
      | PID gain of current controller
      |  P: 0.002
      |  I: 0.00005
      |  D: 0
      | Changing the PID gains is not permitted.
      mask DialogControl ParameterGroupVar Prompt: パラメーター
      mask Display:
      | image('roller485_matlab_fcn.png', [55,10,75,56]);
      | color('orange');
      | text(10, 60, 'current control');
      | text(17, 22, '# mode setting');
      | 
      | color('red');
      | addr = get_param(gcb, 'I2CAddress');
      | text(17, 48, ['I2C: ' addr]);
  current command [mA] (using MATLAB Function) : Subsystem  mask(current command [A]){I2CAddress=0x64, set_time=0}
      mask prompts: I2CAddress "I2C Address"; set_time "Set Time"
      mask help:
      | current mode
      | If t ≤ set_time, then current mode is set.
      | ---------------------------------
      | PID gain of current controller
      |  P: 0.002
      |  I: 0.00005
      |  D: 0
      | Changing the PID gains is not permitted.
      mask DialogControl ParameterGroupVar Prompt: パラメーター
      mask Display:
      | image('roller485_matlab_fcn.png', [55,10,75,56]);
      | color('orange');
      | text(10, 60, 'current control');
      | text(17, 22, '# mode setting');
      | 
      | color('red');
      | addr = get_param(gcb, 'I2CAddress');
      | text(17, 48, ['I2C: ' addr]);
  relative angle command [deg] (using MATLAB Function) : Subsystem  mask(relative angle command [deg]){I2CAddress=0x64, sample_time=0.005, position_P=15, position_I=0.000003, position_D=400, set_time1=0, set_time2=0}
      mask prompts: I2CAddress "I2C Address"; sample_time "Sample Time"; position_P "P"; position_I "I"; position_D "D"; set_time1 "Set Time1"; set_time2 "Set Time2"
      mask help:
      | position mode
      | If t ≤ set_time1, then position mode and initial angle are set.
      | ---------------------------------
      | default value (PID gain of position controller)
      |  P: 15
      |  I: 0.000003
      |  D: 400
      | If t ≤ set_time2, then PID gain can be set.
      mask DialogControl ParameterGroupVar Prompt: パラメーター
      mask Display:
      | image('roller485_matlab_fcn.png', [55,10,75,56]);
      | color('blue');
      | text(10, 60, 'relative position control');
      | text(17, 22, '# mode setting');
      | text(17, 10, '# PID gain setting');
      | 
      | color('red');
      | addr = get_param(gcb, 'I2CAddress');
      | text(17, 48, ['I2C: ' addr]);
  relative angle command [rad] (using MATLAB Function) : Subsystem  mask(relative angle command [rad]){I2CAddress=0x64, sample_time=0.005, position_P=15, position_I=0.000003, position_D=400, set_time1=0, set_time2=0}
      mask prompts: I2CAddress "I2C Address"; sample_time "Sample Time"; position_P "P"; position_I "I"; position_D "D"; set_time1 "Set Time1"; set_time2 "Set Time2"
      mask help:
      | position mode
      | If t ≤ set_time1, then position mode and initial angle are set.
      | ---------------------------------
      | default value (PID gain of position controller)
      |  P: 15
      |  I: 0.000003
      |  D: 400
      | If t ≤ set_time2, then PID gain can be set.
      mask DialogControl ParameterGroupVar Prompt: パラメーター
      mask Display:
      | image('roller485_matlab_fcn.png', [55,10,75,56]);
      | color('blue');
      | text(10, 60, 'relative position control');
      | text(17, 22, '# mode setting');
      | text(17, 10, '# PID gain setting');
      | 
      | color('red');
      | addr = get_param(gcb, 'I2CAddress');
      | text(17, 48, ['I2C: ' addr]);

== system roller485lib/control mode ==
  Data Type Conversion : DataTypeConversion  OutDataTypeStr=uint8  SaturateOnIntegerOverflow=off  RndMeth=Floor
  I2C Write (0x01) : arduinolib/I2C Write  I2CModule=0  Mode=Master  SlaveAddress=I2CAddress  SlaveByteOrder=BigEndian  Direction=Transmitter  RegisterAddressMode=on  RegisterAddress=0x01  SlaveDataType=uint8  DataLength=1  NoAck=off  RepeatedStart=off  OutputStatus=off  blockPlatform=ARDUINO
  mode : Constant  Value=control_mode
  wires:
  Data Type Conversion/1 -> I2C Write (0x01)/1
  mode/1 -> Data Type Conversion/1

== system roller485lib/control mode (initial time only) ==
  Clock : Clock
  Compare To Constant : simulink/Logic and Bit Operations/Compare To Constant  relop===  const=0  OutDataTypeStr=boolean
  Enabled Subsystem : Subsystem  TreatAsAtomicUnit=on
  mode : Constant  Value=control_mode
  wires:
  mode/1 -> Enabled Subsystem/1(mode)
  Compare To Constant/1 -> Enabled Subsystem/Enable
  Clock/1 -> Compare To Constant/1

== system roller485lib/motor ON//OFF ==
  ON (1) or OFF (0) : Inport
  Data Type Conversion : DataTypeConversion  OutDataTypeStr=uint8  SaturateOnIntegerOverflow=off  RndMeth=Floor
  I2C Write (0x00) : arduinolib/I2C Write  I2CModule=0  Mode=Master  SlaveAddress=I2CAddress  SlaveByteOrder=BigEndian  Direction=Transmitter  RegisterAddressMode=on  RegisterAddress=0x00  SlaveDataType=uint8  DataLength=1  NoAck=off  RepeatedStart=off  OutputStatus=off  blockPlatform=ARDUINO
  wires:
  Data Type Conversion/1 -> I2C Write (0x00)/1
  ON (1) or OFF (0)/1 -> Data Type Conversion/1

== system roller485lib/Basic I2C Write/basic absolute angle command [deg] ==
  command [deg] : Inport
  Data Type Conversion : DataTypeConversion  OutDataTypeStr=uint32  SaturateOnIntegerOverflow=off  RndMeth=Floor
  I2C Write (0x80) : arduinolib/I2C Write  I2CModule=0  Mode=Master  SlaveAddress=I2CAddress  SlaveByteOrder=LittleEndian  Direction=Transmitter  RegisterAddressMode=on  RegisterAddress=0x80  SlaveDataType=uint8  DataLength=1  NoAck=off  RepeatedStart=off  OutputStatus=off  blockPlatform=ARDUINO
  x 100 : Gain  Gain=100
  wires:
  command [deg]/1 -> x 100/1
  Data Type Conversion/1 -> I2C Write (0x80)/1
  x 100/1 -> Data Type Conversion/1

== system roller485lib/Basic I2C Write/basic absolute angle command [rad] ==
  command [rad] : Inport
  Data Type Conversion : DataTypeConversion  OutDataTypeStr=uint32  SaturateOnIntegerOverflow=off  RndMeth=Floor
  I2C Write (0x80) : arduinolib/I2C Write  I2CModule=0  Mode=Master  SlaveAddress=I2CAddress  SlaveByteOrder=LittleEndian  Direction=Transmitter  RegisterAddressMode=on  RegisterAddress=0x80  SlaveDataType=uint8  DataLength=1  NoAck=off  RepeatedStart=off  OutputStatus=off  blockPlatform=ARDUINO
  rad to deg : Gain  Gain=180/pi
  x 100 : Gain  Gain=100
  wires:
  command [rad]/1 -> rad to deg/1
  rad to deg/1 -> x 100/1
  Data Type Conversion/1 -> I2C Write (0x80)/1
  x 100/1 -> Data Type Conversion/1
